simulink model "robustpid"  (R2016b)
settings: Solver=ode4  StartTime=0.0  StopTime=50  FixedStep=t_step  MaxStep=0.00001  MinStep=0.00000000001  RelTol=1e-3  EnableMultiTasking=on
values from neighbouring files (symbols this model uses):
  a1 = 0.8    [z_trajectory_extension_m.m]
  a2 = 0.8    [z_trajectory_extension_m.m]
  a3 = 0.9    [z_trajectory_extension_m.m]
  a4 = 7    [z_trajectory_extension_m.m]
  a5 = 7    [z_trajectory_extension_m.m]
  a6 = 5    [z_trajectory_extension_m.m]
  b = 10e-6    (= 1e-05)    [z_trajectory_extension_m.m]
  cm = 2.582e-9    (= 2.582e-09)    [z_trajectory_extension_m.m]
  ct = 1.471e-7    (= 1.471e-07)    [z_trajectory_extension_m.m]
  d = 0.3e-6    (= 3e-07)    [z_trajectory_extension_m.m]
  disturbance = 0.1    [z_trajectory_extension_m.m]
  fd = 50/(2*pi)    (= 7.95774715459)    [z_trajectory_extension_m.m]
  g = 9.81    [z_trajectory_extension_m.m]
  Ix = Ixx    (= 0.047)    [z_trajectory_extension_m.m]
  Ixx = 0.047    [z_trajectory_extension_m.m]
  Iy = Iyy    (= 0.047)    [z_trajectory_extension_m.m]
  Iyy = 0.047    [z_trajectory_extension_m.m]
  Iz = Izz    (= 0.094)    [z_trajectory_extension_m.m]
  Izz = 0.094    [z_trajectory_extension_m.m]
  k1 = 1.98    [z_trajectory_extension_m.m]
  k2 = 1.98    [z_trajectory_extension_m.m]
  k3 = 2.78    [z_trajectory_extension_m.m]
  k4 = 5.25    [z_trajectory_extension_m.m]
  k5 = 5.25    [z_trajectory_extension_m.m]
  k6 = 2.75    [z_trajectory_extension_m.m]
  Kd_phi = 20.5    [z_trajectory_extension_m.m]
  Kd_psi = 20    [z_trajectory_extension_m.m]
  Kd_theta = 20.5    [z_trajectory_extension_m.m]
  Kd_x = 0.5005    [z_trajectory_extension_m.m]
  Kd_y = 0.5005    [z_trajectory_extension_m.m]
  Kd_z = 40.7    [z_trajectory_extension_m.m]
  Ki_phi = 0.001    [z_trajectory_extension_m.m]
  Ki_psi = 0.001    [z_trajectory_extension_m.m]
  Ki_theta = 0.001    [z_trajectory_extension_m.m]
  Ki_x = 0.00    (= 0)    [z_trajectory_extension_m.m]
  Ki_y = 0.00    (= 0)    [z_trajectory_extension_m.m]
  Ki_z = 0.4    [z_trajectory_extension_m.m]
  Kp_phi = 90.0    (= 90)    [z_trajectory_extension_m.m]
  Kp_psi = 50    [z_trajectory_extension_m.m]
  Kp_theta = 90.0    (= 90)    [z_trajectory_extension_m.m]
  Kp_x = 0.5005    [z_trajectory_extension_m.m]
  Kp_y = 0.5005    [z_trajectory_extension_m.m]
  Kp_z = 22.1    [z_trajectory_extension_m.m]
  L = 0.225    [z_trajectory_extension_m.m]
  l1 = 0.9    [z_trajectory_extension_m.m]
  l2 = 0.9    [z_trajectory_extension_m.m]
  l3 = 1.25    [z_trajectory_extension_m.m]
  l4 = 3.5    [z_trajectory_extension_m.m]
  l5 = 3.5    [z_trajectory_extension_m.m]
  l6 = 1.8    [z_trajectory_extension_m.m]
  m = 0.93    [z_trajectory_extension_m.m]
  O = 0.283    [z_trajectory_extension_m.m]
  phi_init = 0    [z_trajectory_extension_m.m]
  phi_ref = 30*3.142/180    (= 0.523666666667)    [z_trajectory_extension_m.m]
  psi_init = 0    [z_trajectory_extension_m.m]
  psi_ref = 20*3.142/180    (= 0.349111111111)    [z_trajectory_extension_m.m]
  smc = 0    [z_trajectory_extension_m.m]
  tau_att = 2    [z_trajectory_extension_m.m]
  tau_att_1 = 2    [z_trajectory_extension_m.m]
  tau_p = 2    [z_trajectory_extension_m.m]
  theta_init = 0    [z_trajectory_extension_m.m]
  theta_ref = 30*3.142/180    (= 0.523666666667)    [z_trajectory_extension_m.m]
  w_lim = 6000    [z_trajectory_extension_m.m]
  xref = 5    [z_trajectory_extension_m.m]
  yref = 15    [z_trajectory_extension_m.m]
  z_inti = 0    [z_trajectory_extension_m.m]
  z_ref = 15    [z_trajectory_extension_m.m]
libraries: simulink x2
(part 2 of 2)

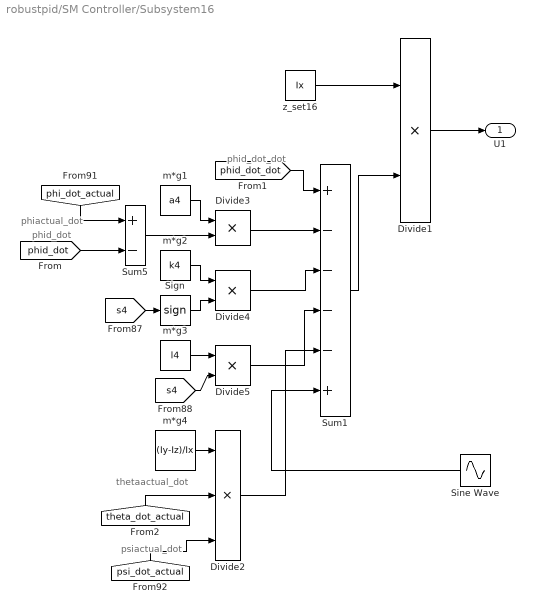
== system robustpid/SM Controller/Subsystem16 ==
  note: psiactual_dot
  note: thetaactual_dot
  note: phid_dot_dot
  note: phid_dot
  note: phiactual_dot
  Divide{1,3..5} (4 alike) : Product  Inputs=**
  Divide2 : Product  Inputs=***
  Sign : Signum
  Sine Wave : Sin  Amplitude=disturbance  Frequency=fd  SampleTime=0
  Sum1 : Sum  Inputs=+----+
  Sum5 : Sum  Inputs=+-
  m*g1 : Constant  Value=a4
  m*g2 : Constant  Value=k4
  m*g3 : Constant  Value=l4
  m*g4 : Constant  Value=(Iy-Iz)/Ix
  z_set16 : Constant  Value=Ix
  U1 : Outport
  wires:
  Divide4/1 -> Sum1/3
  Divide3/1 -> Sum1/2
  m*g1/1 -> Divide3/1
  [s4] -> Sign/1
  [s4] -> Divide5/2
  Sum5/1 -> Divide3/2
  Divide1/1 -> U1/1
  z_set16/1 -> Divide1/1
  Divide5/1 -> Sum1/4
  Sign/1 -> Divide4/2
  m*g3/1 -> Divide5/1
  Sum1/1 -> Divide1/2
  [phid_dot_dot] -> Sum1/1
  [phid_dot] -> Sum5/2
  [phi_dot_actual] -> Sum5/1
  m*g2/1 -> Divide4/1
  Divide2/1 -> Sum1/5
  [theta_dot_actual] -> Divide2/2
  m*g4/1 -> Divide2/1
  [psi_dot_actual] -> Divide2/3
  Sine Wave/1 -> Sum1/6

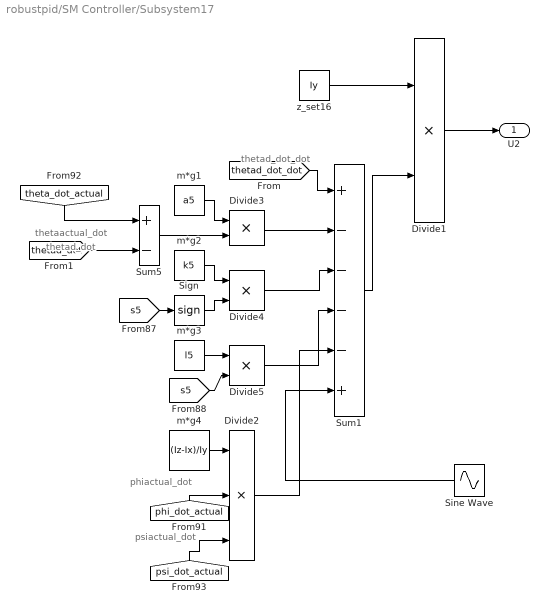
== system robustpid/SM Controller/Subsystem17 ==
  note: thetaactual_dot
  note: thetad_dot
  note: thetad_dot_dot
  note: phiactual_dot
  note: psiactual_dot
  Divide{1,3..5} (4 alike) : Product  Inputs=**
  Divide2 : Product  Inputs=***
  Sign : Signum
  Sine Wave : Sin  Amplitude=disturbance  Frequency=fd  SampleTime=0
  Sum1 : Sum  Inputs=+----+
  Sum5 : Sum  Inputs=+-
  m*g1 : Constant  Value=a5
  m*g2 : Constant  Value=k5
  m*g3 : Constant  Value=l5
  m*g4 : Constant  Value=(Iz-Ix)/Iy
  z_set16 : Constant  Value=Iy
  U2 : Outport
  wires:
  [psi_dot_actual] -> Divide2/3
  m*g4/1 -> Divide2/1
  [phi_dot_actual] -> Divide2/2
  Divide2/1 -> Sum1/5
  m*g2/1 -> Divide4/1
  [theta_dot_actual] -> Sum5/1
  [thetad_dot] -> Sum5/2
  [thetad_dot_dot] -> Sum1/1
  Sum1/1 -> Divide1/2
  m*g3/1 -> Divide5/1
  Sign/1 -> Divide4/2
  Divide5/1 -> Sum1/4
  z_set16/1 -> Divide1/1
  Divide1/1 -> U2/1
  Sum5/1 -> Divide3/2
  [s5] -> Divide5/2
  [s5] -> Sign/1
  m*g1/1 -> Divide3/1
  Divide3/1 -> Sum1/2
  Divide4/1 -> Sum1/3
  Sine Wave/1 -> Sum1/6

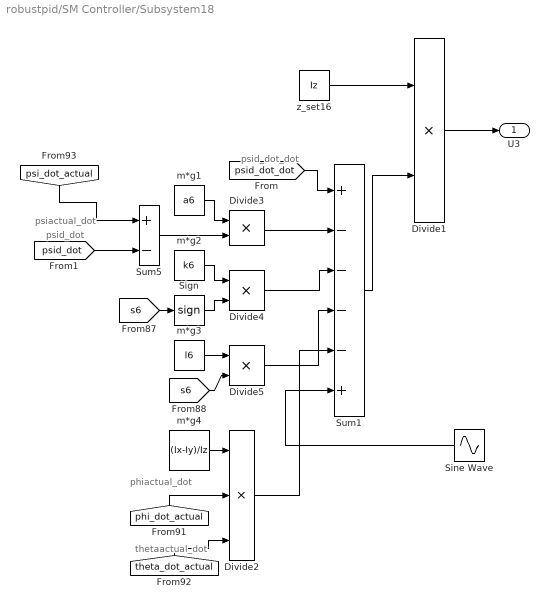
== system robustpid/SM Controller/Subsystem18 ==
  note: thetaactual_dot
  note: phiactual_dot
  note: psid_dot_dot
  note: psid_dot
  note: psiactual_dot
  Divide{1,3..5} (4 alike) : Product  Inputs=**
  Divide2 : Product  Inputs=***
  Sign : Signum
  Sine Wave : Sin  Amplitude=disturbance  Frequency=fd  SampleTime=0
  Sum1 : Sum  Inputs=+----+
  Sum5 : Sum  Inputs=+-
  m*g1 : Constant  Value=a6
  m*g2 : Constant  Value=k6
  m*g3 : Constant  Value=l6
  m*g4 : Constant  Value=(Ix-Iy)/Iz
  z_set16 : Constant  Value=Iz
  U3 : Outport
  wires:
  Divide4/1 -> Sum1/3
  Divide3/1 -> Sum1/2
  m*g1/1 -> Divide3/1
  [s6] -> Sign/1
  [s6] -> Divide5/2
  Sum5/1 -> Divide3/2
  Divide1/1 -> U3/1
  z_set16/1 -> Divide1/1
  Divide5/1 -> Sum1/4
  Sign/1 -> Divide4/2
  m*g3/1 -> Divide5/1
  Sum1/1 -> Divide1/2
  [psid_dot_dot] -> Sum1/1
  [psid_dot] -> Sum5/2
  [psi_dot_actual] -> Sum5/1
  m*g2/1 -> Divide4/1
  Divide2/1 -> Sum1/5
  [phi_dot_actual] -> Divide2/2
  m*g4/1 -> Divide2/1
  [theta_dot_actual] -> Divide2/3
  Sine Wave/1 -> Sum1/6

== system robustpid/SM Controller/Subsystem19 ==
  note: yd_dot
  Divide6 : Product  Inputs=**
  Sum6 : Sum  Inputs=+-+
  Sum7 : Sum  Inputs=+-
  m*g4 : Constant  Value=a4
  s4 : Outport
  wires:
  Sum6/1 -> s4/1
  Divide6/1 -> Sum6/3
  [phi_actual] -> Sum7/1
  [phi_dot_actual] -> Sum6/1
  m*g4/1 -> Divide6/1
  Sum7/1 -> Divide6/2
  [phi_set] -> Sum7/2
  [phid_dot] -> Sum6/2

== system robustpid/SM Controller/Subsystem20 ==
  note: yd_dot
  Divide6 : Product  Inputs=**
  Sum6 : Sum  Inputs=+-+
  Sum7 : Sum  Inputs=+-
  m*g4 : Constant  Value=a5
  s5 : Outport
  wires:
  [thetad_dot] -> Sum6/2
  [theta_set] -> Sum7/2
  Sum7/1 -> Divide6/2
  m*g4/1 -> Divide6/1
  [theta_dot_actual] -> Sum6/1
  [theta_actual] -> Sum7/1
  Divide6/1 -> Sum6/3
  Sum6/1 -> s5/1

== system robustpid/SM Controller/Subsystem21 ==
  note: yd_dot
  Divide6 : Product  Inputs=**
  Sum6 : Sum  Inputs=+-+
  Sum7 : Sum  Inputs=+-
  m*g4 : Constant  Value=a6
  pitch_TF : TransferFcn  Commented=on  Denominator=[tau_att 1]
  z_set3 : Constant  Value=psi_ref
  s6 : Outport
  wires:
  Sum6/1 -> s6/1
  Divide6/1 -> Sum6/3
  [psi_actual] -> Sum7/1
  [psi_dot_actual] -> Sum6/1
  m*g4/1 -> Divide6/1
  Sum7/1 -> Divide6/2
  z_set3/1 -> Sum7/2, pitch_TF/1
  [psid_dot] -> Sum6/2
